simulink model "elevator"  (R2020a)
settings: Solver=VariableStepAuto  StartTime=0.0  StopTime=inf  RelTol=1e-3
PreLoadFcn:
  | slplc.api.loadDataTypes;
undefined symbols (not defined in the file): BOOL, DINT, INT, slplc
libraries: simulink x1
(part 38 of 38)

== matlab function elevator/PLCControllerSuite/__Logic/Task/Program/__Logic/XIC46/__Format ==
  data: BlockEnable input; RungIn input; RungOut input; data input
function setBlockFormat(BlockEnable, RungIn, RungOut, data)

if data~=0 && data~=1
    error('slplc:inivalidBooleanValue', 'Invalid boolean value %d', data);
end
data = logical(data);

% set parent block colors
coder.extrinsic('slplc.utils.setBlockAppearance');
persistent lastBlockEnable lastRungIn lastRungOut lastData isInit lastAnimation lastDataShow;
if isempty(lastBlockEnable)
    lastBlockEnable = true;
end
if isempty(lastRungIn)
    lastRungIn = false;
end
if isempty(lastRungOut)
    lastRungOut = false;
end
if isempty(lastData)
    lastData = data;
end
if isempty(isInit)
    isInit = true;
else
    isInit = false;
end
if isempty(lastAnimation)
    lastAnimation = false;
end
if isempty(lastDataShow)
    lastDataShow = false;
end

[animation, dataShow] = slplc.utils.setBlockAppearance('set', '%<PLCOperandTag>', {}, {}, ...
    ' = ', {'ForegroundColor'}, ...
    isInit,  ...
    BlockEnable, lastBlockEnable, ...
    RungIn,  lastRungIn, ...
    RungOut, lastRungOut, ...
    data, lastData, ...
    lastAnimation, lastDataShow);

lastBlockEnable = BlockEnable;
lastRungIn      = RungIn;
lastRungOut     = RungOut;
lastData        = data;
lastAnimation   = animation;
lastDataShow    = dataShow;
end

== matlab function elevator/PLCControllerSuite/__Logic/Task/Program/__Logic/Junction1/__Format ==
  data: BlockEnable input; RungOut input
function setBlockFormat(BlockEnable, RungOut)
% set parent block colors
coder.extrinsic('slplc.utils.setBlockAppearance');
persistent lastBlockEnable isInit lastRungOut lastAnimation lastRungOutShow;
if isempty(lastBlockEnable)
    lastBlockEnable = true;
end

if isempty(isInit)
    isInit = true;
else
    isInit = false;
end

if isempty(lastRungOut)
    lastRungOut = RungOut;
end

if isempty(lastAnimation)
    lastAnimation = false;
end

if isempty(lastRungOutShow)
    lastRungOutShow = false;
end

[animation, dataShow] = slplc.utils.setBlockAppearance('set', '', {'black', 'black'}, {}, ...
    '', {'ForegroundColor', 'BackgroundColor'}, ...
    isInit,  ...
    BlockEnable, lastBlockEnable, ...
    RungOut,   lastRungOut, ...
    RungOut,   lastRungOut, ...
    [],    [], ...
    lastAnimation, lastRungOutShow);

lastBlockEnable     = BlockEnable;
lastRungOut         = RungOut;
lastAnimation       = animation;
lastRungOutShow     = dataShow;
end

== matlab function elevator/PLCControllerSuite/__Logic/Task/Program/__Logic/XIC47/__Format ==
  data: BlockEnable input; RungIn input; RungOut input; data input
function setBlockFormat(BlockEnable, RungIn, RungOut, data)

if data~=0 && data~=1
    error('slplc:inivalidBooleanValue', 'Invalid boolean value %d', data);
end
data = logical(data);

% set parent block colors
coder.extrinsic('slplc.utils.setBlockAppearance');
persistent lastBlockEnable lastRungIn lastRungOut lastData isInit lastAnimation lastDataShow;
if isempty(lastBlockEnable)
    lastBlockEnable = true;
end
if isempty(lastRungIn)
    lastRungIn = false;
end
if isempty(lastRungOut)
    lastRungOut = false;
end
if isempty(lastData)
    lastData = data;
end
if isempty(isInit)
    isInit = true;
else
    isInit = false;
end
if isempty(lastAnimation)
    lastAnimation = false;
end
if isempty(lastDataShow)
    lastDataShow = false;
end

[animation, dataShow] = slplc.utils.setBlockAppearance('set', '%<PLCOperandTag>', {}, {}, ...
    ' = ', {'ForegroundColor'}, ...
    isInit,  ...
    BlockEnable, lastBlockEnable, ...
    RungIn,  lastRungIn, ...
    RungOut, lastRungOut, ...
    data, lastData, ...
    lastAnimation, lastDataShow);

lastBlockEnable = BlockEnable;
lastRungIn      = RungIn;
lastRungOut     = RungOut;
lastData        = data;
lastAnimation   = animation;
lastDataShow    = dataShow;
end

== matlab function elevator/PLCControllerSuite/__Logic/Task/Program/__Logic/XIC48/__Format ==
  data: BlockEnable input; RungIn input; RungOut input; data input
function setBlockFormat(BlockEnable, RungIn, RungOut, data)

if data~=0 && data~=1
    error('slplc:inivalidBooleanValue', 'Invalid boolean value %d', data);
end
data = logical(data);

% set parent block colors
coder.extrinsic('slplc.utils.setBlockAppearance');
persistent lastBlockEnable lastRungIn lastRungOut lastData isInit lastAnimation lastDataShow;
if isempty(lastBlockEnable)
    lastBlockEnable = true;
end
if isempty(lastRungIn)
    lastRungIn = false;
end
if isempty(lastRungOut)
    lastRungOut = false;
end
if isempty(lastData)
    lastData = data;
end
if isempty(isInit)
    isInit = true;
else
    isInit = false;
end
if isempty(lastAnimation)
    lastAnimation = false;
end
if isempty(lastDataShow)
    lastDataShow = false;
end

[animation, dataShow] = slplc.utils.setBlockAppearance('set', '%<PLCOperandTag>', {}, {}, ...
    ' = ', {'ForegroundColor'}, ...
    isInit,  ...
    BlockEnable, lastBlockEnable, ...
    RungIn,  lastRungIn, ...
    RungOut, lastRungOut, ...
    data, lastData, ...
    lastAnimation, lastDataShow);

lastBlockEnable = BlockEnable;
lastRungIn      = RungIn;
lastRungOut     = RungOut;
lastData        = data;
lastAnimation   = animation;
lastDataShow    = dataShow;
end

== matlab function elevator/PLCControllerSuite/__Logic/Task/Program/__Logic/XIC49/__Format ==
  data: BlockEnable input; RungIn input; RungOut input; data input
function setBlockFormat(BlockEnable, RungIn, RungOut, data)

if data~=0 && data~=1
    error('slplc:inivalidBooleanValue', 'Invalid boolean value %d', data);
end
data = logical(data);

% set parent block colors
coder.extrinsic('slplc.utils.setBlockAppearance');
persistent lastBlockEnable lastRungIn lastRungOut lastData isInit lastAnimation lastDataShow;
if isempty(lastBlockEnable)
    lastBlockEnable = true;
end
if isempty(lastRungIn)
    lastRungIn = false;
end
if isempty(lastRungOut)
    lastRungOut = false;
end
if isempty(lastData)
    lastData = data;
end
if isempty(isInit)
    isInit = true;
else
    isInit = false;
end
if isempty(lastAnimation)
    lastAnimation = false;
end
if isempty(lastDataShow)
    lastDataShow = false;
end

[animation, dataShow] = slplc.utils.setBlockAppearance('set', '%<PLCOperandTag>', {}, {}, ...
    ' = ', {'ForegroundColor'}, ...
    isInit,  ...
    BlockEnable, lastBlockEnable, ...
    RungIn,  lastRungIn, ...
    RungOut, lastRungOut, ...
    data, lastData, ...
    lastAnimation, lastDataShow);

lastBlockEnable = BlockEnable;
lastRungIn      = RungIn;
lastRungOut     = RungOut;
lastData        = data;
lastAnimation   = animation;
lastDataShow    = dataShow;
end

== matlab function elevator/PLCControllerSuite/__Logic/Task/Program/__Logic/XIC50/__Format ==
  data: BlockEnable input; RungIn input; RungOut input; data input
function setBlockFormat(BlockEnable, RungIn, RungOut, data)

if data~=0 && data~=1
    error('slplc:inivalidBooleanValue', 'Invalid boolean value %d', data);
end
data = logical(data);

% set parent block colors
coder.extrinsic('slplc.utils.setBlockAppearance');
persistent lastBlockEnable lastRungIn lastRungOut lastData isInit lastAnimation lastDataShow;
if isempty(lastBlockEnable)
    lastBlockEnable = true;
end
if isempty(lastRungIn)
    lastRungIn = false;
end
if isempty(lastRungOut)
    lastRungOut = false;
end
if isempty(lastData)
    lastData = data;
end
if isempty(isInit)
    isInit = true;
else
    isInit = false;
end
if isempty(lastAnimation)
    lastAnimation = false;
end
if isempty(lastDataShow)
    lastDataShow = false;
end

[animation, dataShow] = slplc.utils.setBlockAppearance('set', '%<PLCOperandTag>', {}, {}, ...
    ' = ', {'ForegroundColor'}, ...
    isInit,  ...
    BlockEnable, lastBlockEnable, ...
    RungIn,  lastRungIn, ...
    RungOut, lastRungOut, ...
    data, lastData, ...
    lastAnimation, lastDataShow);

lastBlockEnable = BlockEnable;
lastRungIn      = RungIn;
lastRungOut     = RungOut;
lastData        = data;
lastAnimation   = animation;
lastDataShow    = dataShow;
end

== matlab function elevator/PLCControllerSuite/__Logic/Task/Program/__Logic/XIC51/__Format ==
  data: BlockEnable input; RungIn input; RungOut input; data input
function setBlockFormat(BlockEnable, RungIn, RungOut, data)

if data~=0 && data~=1
    error('slplc:inivalidBooleanValue', 'Invalid boolean value %d', data);
end
data = logical(data);

% set parent block colors
coder.extrinsic('slplc.utils.setBlockAppearance');
persistent lastBlockEnable lastRungIn lastRungOut lastData isInit lastAnimation lastDataShow;
if isempty(lastBlockEnable)
    lastBlockEnable = true;
end
if isempty(lastRungIn)
    lastRungIn = false;
end
if isempty(lastRungOut)
    lastRungOut = false;
end
if isempty(lastData)
    lastData = data;
end
if isempty(isInit)
    isInit = true;
else
    isInit = false;
end
if isempty(lastAnimation)
    lastAnimation = false;
end
if isempty(lastDataShow)
    lastDataShow = false;
end

[animation, dataShow] = slplc.utils.setBlockAppearance('set', '%<PLCOperandTag>', {}, {}, ...
    ' = ', {'ForegroundColor'}, ...
    isInit,  ...
    BlockEnable, lastBlockEnable, ...
    RungIn,  lastRungIn, ...
    RungOut, lastRungOut, ...
    data, lastData, ...
    lastAnimation, lastDataShow);

lastBlockEnable = BlockEnable;
lastRungIn      = RungIn;
lastRungOut     = RungOut;
lastData        = data;
lastAnimation   = animation;
lastDataShow    = dataShow;
end

== matlab function elevator/PLCControllerSuite/__Logic/Task/Program/__Logic/XIC52/__Format ==
  data: BlockEnable input; RungIn input; RungOut input; data input
function setBlockFormat(BlockEnable, RungIn, RungOut, data)

if data~=0 && data~=1
    error('slplc:inivalidBooleanValue', 'Invalid boolean value %d', data);
end
data = logical(data);

% set parent block colors
coder.extrinsic('slplc.utils.setBlockAppearance');
persistent lastBlockEnable lastRungIn lastRungOut lastData isInit lastAnimation lastDataShow;
if isempty(lastBlockEnable)
    lastBlockEnable = true;
end
if isempty(lastRungIn)
    lastRungIn = false;
end
if isempty(lastRungOut)
    lastRungOut = false;
end
if isempty(lastData)
    lastData = data;
end
if isempty(isInit)
    isInit = true;
else
    isInit = false;
end
if isempty(lastAnimation)
    lastAnimation = false;
end
if isempty(lastDataShow)
    lastDataShow = false;
end

[animation, dataShow] = slplc.utils.setBlockAppearance('set', '%<PLCOperandTag>', {}, {}, ...
    ' = ', {'ForegroundColor'}, ...
    isInit,  ...
    BlockEnable, lastBlockEnable, ...
    RungIn,  lastRungIn, ...
    RungOut, lastRungOut, ...
    data, lastData, ...
    lastAnimation, lastDataShow);

lastBlockEnable = BlockEnable;
lastRungIn      = RungIn;
lastRungOut     = RungOut;
lastData        = data;
lastAnimation   = animation;
lastDataShow    = dataShow;
end

== matlab function elevator/PLCControllerSuite/__Logic/Task/Program/__Logic/XIC53/__Format ==
  data: BlockEnable input; RungIn input; RungOut input; data input
function setBlockFormat(BlockEnable, RungIn, RungOut, data)

if data~=0 && data~=1
    error('slplc:inivalidBooleanValue', 'Invalid boolean value %d', data);
end
data = logical(data);

% set parent block colors
coder.extrinsic('slplc.utils.setBlockAppearance');
persistent lastBlockEnable lastRungIn lastRungOut lastData isInit lastAnimation lastDataShow;
if isempty(lastBlockEnable)
    lastBlockEnable = true;
end
if isempty(lastRungIn)
    lastRungIn = false;
end
if isempty(lastRungOut)
    lastRungOut = false;
end
if isempty(lastData)
    lastData = data;
end
if isempty(isInit)
    isInit = true;
else
    isInit = false;
end
if isempty(lastAnimation)
    lastAnimation = false;
end
if isempty(lastDataShow)
    lastDataShow = false;
end

[animation, dataShow] = slplc.utils.setBlockAppearance('set', '%<PLCOperandTag>', {}, {}, ...
    ' = ', {'ForegroundColor'}, ...
    isInit,  ...
    BlockEnable, lastBlockEnable, ...
    RungIn,  lastRungIn, ...
    RungOut, lastRungOut, ...
    data, lastData, ...
    lastAnimation, lastDataShow);

lastBlockEnable = BlockEnable;
lastRungIn      = RungIn;
lastRungOut     = RungOut;
lastData        = data;
lastAnimation   = animation;
lastDataShow    = dataShow;
end

== matlab function elevator/PLCControllerSuite/__Logic/Task/Program/__Logic/XIC54/__Format ==
  data: BlockEnable input; RungIn input; RungOut input; data input
function setBlockFormat(BlockEnable, RungIn, RungOut, data)

if data~=0 && data~=1
    error('slplc:inivalidBooleanValue', 'Invalid boolean value %d', data);
end
data = logical(data);

% set parent block colors
coder.extrinsic('slplc.utils.setBlockAppearance');
persistent lastBlockEnable lastRungIn lastRungOut lastData isInit lastAnimation lastDataShow;
if isempty(lastBlockEnable)
    lastBlockEnable = true;
end
if isempty(lastRungIn)
    lastRungIn = false;
end
if isempty(lastRungOut)
    lastRungOut = false;
end
if isempty(lastData)
    lastData = data;
end
if isempty(isInit)
    isInit = true;
else
    isInit = false;
end
if isempty(lastAnimation)
    lastAnimation = false;
end
if isempty(lastDataShow)
    lastDataShow = false;
end

[animation, dataShow] = slplc.utils.setBlockAppearance('set', '%<PLCOperandTag>', {}, {}, ...
    ' = ', {'ForegroundColor'}, ...
    isInit,  ...
    BlockEnable, lastBlockEnable, ...
    RungIn,  lastRungIn, ...
    RungOut, lastRungOut, ...
    data, lastData, ...
    lastAnimation, lastDataShow);

lastBlockEnable = BlockEnable;
lastRungIn      = RungIn;
lastRungOut     = RungOut;
lastData        = data;
lastAnimation   = animation;
lastDataShow    = dataShow;
end

== matlab function elevator/PLCControllerSuite/__Logic/Task/Program/__Logic/XIC4/__Format ==
  data: BlockEnable input; RungIn input; RungOut input; data input
function setBlockFormat(BlockEnable, RungIn, RungOut, data)

if data~=0 && data~=1
    error('slplc:inivalidBooleanValue', 'Invalid boolean value %d', data);
end
data = logical(data);

% set parent block colors
coder.extrinsic('slplc.utils.setBlockAppearance');
persistent lastBlockEnable lastRungIn lastRungOut lastData isInit lastAnimation lastDataShow;
if isempty(lastBlockEnable)
    lastBlockEnable = true;
end
if isempty(lastRungIn)
    lastRungIn = false;
end
if isempty(lastRungOut)
    lastRungOut = false;
end
if isempty(lastData)
    lastData = data;
end
if isempty(isInit)
    isInit = true;
else
    isInit = false;
end
if isempty(lastAnimation)
    lastAnimation = false;
end
if isempty(lastDataShow)
    lastDataShow = false;
end

[animation, dataShow] = slplc.utils.setBlockAppearance('set', '%<PLCOperandTag>', {}, {}, ...
    ' = ', {'ForegroundColor'}, ...
    isInit,  ...
    BlockEnable, lastBlockEnable, ...
    RungIn,  lastRungIn, ...
    RungOut, lastRungOut, ...
    data, lastData, ...
    lastAnimation, lastDataShow);

lastBlockEnable = BlockEnable;
lastRungIn      = RungIn;
lastRungOut     = RungOut;
lastData        = data;
lastAnimation   = animation;
lastDataShow    = dataShow;
end

== matlab function elevator/PLCControllerSuite/__Logic/Task/Program/__Logic/XIC55/__Format ==
  data: BlockEnable input; RungIn input; RungOut input; data input
function setBlockFormat(BlockEnable, RungIn, RungOut, data)

if data~=0 && data~=1
    error('slplc:inivalidBooleanValue', 'Invalid boolean value %d', data);
end
data = logical(data);

% set parent block colors
coder.extrinsic('slplc.utils.setBlockAppearance');
persistent lastBlockEnable lastRungIn lastRungOut lastData isInit lastAnimation lastDataShow;
if isempty(lastBlockEnable)
    lastBlockEnable = true;
end
if isempty(lastRungIn)
    lastRungIn = false;
end
if isempty(lastRungOut)
    lastRungOut = false;
end
if isempty(lastData)
    lastData = data;
end
if isempty(isInit)
    isInit = true;
else
    isInit = false;
end
if isempty(lastAnimation)
    lastAnimation = false;
end
if isempty(lastDataShow)
    lastDataShow = false;
end

[animation, dataShow] = slplc.utils.setBlockAppearance('set', '%<PLCOperandTag>', {}, {}, ...
    ' = ', {'ForegroundColor'}, ...
    isInit,  ...
    BlockEnable, lastBlockEnable, ...
    RungIn,  lastRungIn, ...
    RungOut, lastRungOut, ...
    data, lastData, ...
    lastAnimation, lastDataShow);

lastBlockEnable = BlockEnable;
lastRungIn      = RungIn;
lastRungOut     = RungOut;
lastData        = data;
lastAnimation   = animation;
lastDataShow    = dataShow;
end

== matlab function elevator/PLCControllerSuite/__Logic/Task/Program/__Logic/XIC56/__Format ==
  data: BlockEnable input; RungIn input; RungOut input; data input
function setBlockFormat(BlockEnable, RungIn, RungOut, data)

if data~=0 && data~=1
    error('slplc:inivalidBooleanValue', 'Invalid boolean value %d', data);
end
data = logical(data);

% set parent block colors
coder.extrinsic('slplc.utils.setBlockAppearance');
persistent lastBlockEnable lastRungIn lastRungOut lastData isInit lastAnimation lastDataShow;
if isempty(lastBlockEnable)
    lastBlockEnable = true;
end
if isempty(lastRungIn)
    lastRungIn = false;
end
if isempty(lastRungOut)
    lastRungOut = false;
end
if isempty(lastData)
    lastData = data;
end
if isempty(isInit)
    isInit = true;
else
    isInit = false;
end
if isempty(lastAnimation)
    lastAnimation = false;
end
if isempty(lastDataShow)
    lastDataShow = false;
end

[animation, dataShow] = slplc.utils.setBlockAppearance('set', '%<PLCOperandTag>', {}, {}, ...
    ' = ', {'ForegroundColor'}, ...
    isInit,  ...
    BlockEnable, lastBlockEnable, ...
    RungIn,  lastRungIn, ...
    RungOut, lastRungOut, ...
    data, lastData, ...
    lastAnimation, lastDataShow);

lastBlockEnable = BlockEnable;
lastRungIn      = RungIn;
lastRungOut     = RungOut;
lastData        = data;
lastAnimation   = animation;
lastDataShow    = dataShow;
end

== matlab function elevator/PLCControllerSuite/__Logic/Task/Program/__Logic/XIO27/__Format ==
  data: BlockEnable input; RungIn input; RungOut input; data input
function setBlockFormat(BlockEnable, RungIn, RungOut, data)

if data~=0 && data~=1
    error('slplc:inivalidBooleanValue', 'Invalid boolean value %d', data);
end
data = logical(data);

% set parent block colors
coder.extrinsic('slplc.utils.setBlockAppearance');
persistent lastBlockEnable lastRungIn lastRungOut lastData isInit lastAnimation lastDataShow;
if isempty(lastBlockEnable)
    lastBlockEnable = true;
end
if isempty(lastRungIn)
    lastRungIn = false;
end
if isempty(lastRungOut)
    lastRungOut = false;
end
if isempty(lastData)
    lastData = data;
end
if isempty(isInit)
    isInit = true;
else
    isInit = false;
end
if isempty(lastAnimation)
    lastAnimation = false;
end
if isempty(lastDataShow)
    lastDataShow = false;
end

[animation, dataShow] = slplc.utils.setBlockAppearance('set', '%<PLCOperandTag>', {}, {}, ...
    ' = ', {'ForegroundColor'}, ...
    isInit,  ...
    BlockEnable, lastBlockEnable, ...
    RungIn,  lastRungIn, ...
    RungOut, lastRungOut, ...
    data, lastData, ...
    lastAnimation, lastDataShow);

lastBlockEnable = BlockEnable;
lastRungIn      = RungIn;
lastRungOut     = RungOut;
lastData        = data;
lastAnimation   = animation;
lastDataShow    = dataShow;
end

== matlab function elevator/PLCControllerSuite/__Logic/Task/Program/__Logic/OTE8/__Format ==
  data: BlockEnable input; RungIn input; RungOut input; data input
function setBlockFormat(BlockEnable, RungIn, RungOut, data)

if data~=0 && data~=1
    error('slplc:inivalidBooleanValue', 'Invalid boolean value %d', data);
end
data = logical(data);

% set parent block colors
coder.extrinsic('slplc.utils.setBlockAppearance');
persistent lastBlockEnable lastRungIn lastRungOut lastData isInit lastAnimation lastDataShow;
if isempty(lastBlockEnable)
    lastBlockEnable = true;
end
if isempty(lastRungIn)
    lastRungIn = false;
end
if isempty(lastRungOut)
    lastRungOut = false;
end
if isempty(lastData)
    lastData = data;
end
if isempty(isInit)
    isInit = true;
else
    isInit = false;
end
if isempty(lastAnimation)
    lastAnimation = false;
end
if isempty(lastDataShow)
    lastDataShow = false;
end

[animation, dataShow] = slplc.utils.setBlockAppearance('set', '%<PLCOperandTag>', {}, {}, ...
    ' = ', {'ForegroundColor'}, ...
    isInit,  ...
    BlockEnable, lastBlockEnable, ...
    RungIn,  lastRungIn, ...
    RungOut, lastRungOut, ...
    data, lastData, ...
    lastAnimation, lastDataShow);

lastBlockEnable = BlockEnable;
lastRungIn      = RungIn;
lastRungOut     = RungOut;
lastData        = data;
lastAnimation   = animation;
lastDataShow    = dataShow;
end

== matlab function elevator/PLCControllerSuite/__Logic/Task/Program/__Logic/XIC34/__Format ==
  data: BlockEnable input; RungIn input; RungOut input; data input
function setBlockFormat(BlockEnable, RungIn, RungOut, data)

if data~=0 && data~=1
    error('slplc:inivalidBooleanValue', 'Invalid boolean value %d', data);
end
data = logical(data);

% set parent block colors
coder.extrinsic('slplc.utils.setBlockAppearance');
persistent lastBlockEnable lastRungIn lastRungOut lastData isInit lastAnimation lastDataShow;
if isempty(lastBlockEnable)
    lastBlockEnable = true;
end
if isempty(lastRungIn)
    lastRungIn = false;
end
if isempty(lastRungOut)
    lastRungOut = false;
end
if isempty(lastData)
    lastData = data;
end
if isempty(isInit)
    isInit = true;
else
    isInit = false;
end
if isempty(lastAnimation)
    lastAnimation = false;
end
if isempty(lastDataShow)
    lastDataShow = false;
end

[animation, dataShow] = slplc.utils.setBlockAppearance('set', '%<PLCOperandTag>', {}, {}, ...
    ' = ', {'ForegroundColor'}, ...
    isInit,  ...
    BlockEnable, lastBlockEnable, ...
    RungIn,  lastRungIn, ...
    RungOut, lastRungOut, ...
    data, lastData, ...
    lastAnimation, lastDataShow);

lastBlockEnable = BlockEnable;
lastRungIn      = RungIn;
lastRungOut     = RungOut;
lastData        = data;
lastAnimation   = animation;
lastDataShow    = dataShow;
end

== matlab function elevator/PLCControllerSuite/__Logic/Task/Program/__Logic/Variable Write1/__Format ==
  data: data input
function setBlockFormat(data)
% set parent block colors
coder.extrinsic('slplc.utils.setBlockAppearance');
persistent isInit lastData  lastAnimation lastDataShow;

if isempty(isInit)
    isInit = true;
else
    isInit = false;
end

if isempty(lastData)
    lastData = data;
end

if isempty(lastAnimation)
    lastAnimation = false;
end

if isempty(lastDataShow)
    lastDataShow = false;
end

[animation, dataShow] = slplc.utils.setBlockAppearance('set', '', {}, {}, ...
    '%<PLCOperandTag> = ', {}, ...
    isInit,  ...
    true,  true, ...
    false, false, ...
    false, false, ...
    data,  lastData, ...
    lastAnimation, lastDataShow);

lastData        = data;
lastAnimation   = animation;
lastDataShow    = dataShow;
end

== matlab function elevator/PLCControllerSuite/__Logic/Task/Program/__Logic/Variable Write2/__Format ==
  data: data input
function setBlockFormat(data)
% set parent block colors
coder.extrinsic('slplc.utils.setBlockAppearance');
persistent isInit lastData  lastAnimation lastDataShow;

if isempty(isInit)
    isInit = true;
else
    isInit = false;
end

if isempty(lastData)
    lastData = data;
end

if isempty(lastAnimation)
    lastAnimation = false;
end

if isempty(lastDataShow)
    lastDataShow = false;
end

[animation, dataShow] = slplc.utils.setBlockAppearance('set', '', {}, {}, ...
    '%<PLCOperandTag> = ', {}, ...
    isInit,  ...
    true,  true, ...
    false, false, ...
    false, false, ...
    data,  lastData, ...
    lastAnimation, lastDataShow);

lastData        = data;
lastAnimation   = animation;
lastDataShow    = dataShow;
end

== matlab function elevator/PLCControllerSuite/__Logic/Task/Program/__Logic/Variable Write3/__Format ==
  data: data input
function setBlockFormat(data)
% set parent block colors
coder.extrinsic('slplc.utils.setBlockAppearance');
persistent isInit lastData  lastAnimation lastDataShow;

if isempty(isInit)
    isInit = true;
else
    isInit = false;
end

if isempty(lastData)
    lastData = data;
end

if isempty(lastAnimation)
    lastAnimation = false;
end

if isempty(lastDataShow)
    lastDataShow = false;
end

[animation, dataShow] = slplc.utils.setBlockAppearance('set', '', {}, {}, ...
    '%<PLCOperandTag> = ', {}, ...
    isInit,  ...
    true,  true, ...
    false, false, ...
    false, false, ...
    data,  lastData, ...
    lastAnimation, lastDataShow);

lastData        = data;
lastAnimation   = animation;
lastDataShow    = dataShow;
end

== matlab function elevator/PLCControllerSuite/__Logic/Task/Program/__Logic/XIC41/__Format ==
  data: BlockEnable input; RungIn input; RungOut input; data input
function setBlockFormat(BlockEnable, RungIn, RungOut, data)

if data~=0 && data~=1
    error('slplc:inivalidBooleanValue', 'Invalid boolean value %d', data);
end
data = logical(data);

% set parent block colors
coder.extrinsic('slplc.utils.setBlockAppearance');
persistent lastBlockEnable lastRungIn lastRungOut lastData isInit lastAnimation lastDataShow;
if isempty(lastBlockEnable)
    lastBlockEnable = true;
end
if isempty(lastRungIn)
    lastRungIn = false;
end
if isempty(lastRungOut)
    lastRungOut = false;
end
if isempty(lastData)
    lastData = data;
end
if isempty(isInit)
    isInit = true;
else
    isInit = false;
end
if isempty(lastAnimation)
    lastAnimation = false;
end
if isempty(lastDataShow)
    lastDataShow = false;
end

[animation, dataShow] = slplc.utils.setBlockAppearance('set', '%<PLCOperandTag>', {}, {}, ...
    ' = ', {'ForegroundColor'}, ...
    isInit,  ...
    BlockEnable, lastBlockEnable, ...
    RungIn,  lastRungIn, ...
    RungOut, lastRungOut, ...
    data, lastData, ...
    lastAnimation, lastDataShow);

lastBlockEnable = BlockEnable;
lastRungIn      = RungIn;
lastRungOut     = RungOut;
lastData        = data;
lastAnimation   = animation;
lastDataShow    = dataShow;
end

== matlab function elevator/PLCControllerSuite/__Logic/Task/Program/__Logic/TON/Instruction_Enable/__Logic ==
  data: EN output; TT output; RungIn input; PRE input; EN input; DN input; DN output; ACC output; ACC input; currentTime input; lastTime input
function [EN, TT, DN, ACC]  = TON(RungIn, PRE, EN, DN, ACC, currentTime, lastTime)
% TON algorithm

if RungIn
    % Rung-condition-in is True
    if PRE < 0 || ACC < 0
        error('slplc:TONError', '.PRE or .ACC cannot be negtive values');
    end
    TT = true;
    if ~DN
        if EN
            deltaT = currentTime - lastTime;
            ACC = ACC + cast(deltaT, class(ACC));
            if ACC == intmax(class(ACC)) || ACC >= PRE
                TT = false;
                DN = true;
            end
        end
    else
        TT = false;
    end
    EN = true;
    % True end
else
    % Rung-condition-in is False
    EN    = false;
    TT    = false;
    DN    = false;
    ACC   = cast(0, class(ACC));
    % False end
end

end

== matlab function elevator/PLCControllerSuite/__Logic/Task/Program/__Logic/OTE1/__Format ==
  data: BlockEnable input; RungIn input; RungOut input; data input
function setBlockFormat(BlockEnable, RungIn, RungOut, data)

if data~=0 && data~=1
    error('slplc:inivalidBooleanValue', 'Invalid boolean value %d', data);
end
data = logical(data);

% set parent block colors
coder.extrinsic('slplc.utils.setBlockAppearance');
persistent lastBlockEnable lastRungIn lastRungOut lastData isInit lastAnimation lastDataShow;
if isempty(lastBlockEnable)
    lastBlockEnable = true;
end
if isempty(lastRungIn)
    lastRungIn = false;
end
if isempty(lastRungOut)
    lastRungOut = false;
end
if isempty(lastData)
    lastData = data;
end
if isempty(isInit)
    isInit = true;
else
    isInit = false;
end
if isempty(lastAnimation)
    lastAnimation = false;
end
if isempty(lastDataShow)
    lastDataShow = false;
end

[animation, dataShow] = slplc.utils.setBlockAppearance('set', '%<PLCOperandTag>', {}, {}, ...
    ' = ', {'ForegroundColor'}, ...
    isInit,  ...
    BlockEnable, lastBlockEnable, ...
    RungIn,  lastRungIn, ...
    RungOut, lastRungOut, ...
    data, lastData, ...
    lastAnimation, lastDataShow);

lastBlockEnable = BlockEnable;
lastRungIn      = RungIn;
lastRungOut     = RungOut;
lastData        = data;
lastAnimation   = animation;
lastDataShow    = dataShow;
end

== matlab function elevator/PLCControllerSuite/__Logic/Task/Program/__Logic/TON/__Format ==
  data: BlockEnable input; RungIn input; RungOut input; data input
function setBlockFormat(BlockEnable, RungIn, RungOut, data)
% set parent block colors
coder.extrinsic('slplc.utils.setBlockAppearance');
persistent lastBlockEnable lastRungIn lastRungOut lastData isInit lastAnimation lastDataShow;
if isempty(lastBlockEnable)
    lastBlockEnable = true;
end
if isempty(lastRungIn)
    lastRungIn = false;
end
if isempty(lastRungOut)
    lastRungOut = false;
end
if isempty(lastData)
    lastData = data;
end
if isempty(isInit)
    isInit = true;
else
    isInit = false;
end
if isempty(lastAnimation)
    lastAnimation = false;
end
if isempty(lastDataShow)
    lastDataShow = false;
end

[animation, dataShow] = slplc.utils.setBlockAppearance('set', '%<PLCBlockType>: %<PLCOperandTag>', {}, {}, ...
    ' = ', {'ForegroundColor'}, ...
    isInit,  ...
    BlockEnable, lastBlockEnable, ...
    RungIn,  lastRungIn, ...
    RungOut, lastRungOut, ...
    data, lastData, ...
    lastAnimation, lastDataShow);

lastBlockEnable = BlockEnable;
lastRungIn      = RungIn;
lastRungOut     = RungOut;
lastData        = data;
lastAnimation   = animation;
lastDataShow    = dataShow;
end

== matlab function elevator/PLCControllerSuite/__Logic/Task/Program/__Logic/OTE11/__Format ==
  data: BlockEnable input; RungIn input; RungOut input; data input
function setBlockFormat(BlockEnable, RungIn, RungOut, data)

if data~=0 && data~=1
    error('slplc:inivalidBooleanValue', 'Invalid boolean value %d', data);
end
data = logical(data);

% set parent block colors
coder.extrinsic('slplc.utils.setBlockAppearance');
persistent lastBlockEnable lastRungIn lastRungOut lastData isInit lastAnimation lastDataShow;
if isempty(lastBlockEnable)
    lastBlockEnable = true;
end
if isempty(lastRungIn)
    lastRungIn = false;
end
if isempty(lastRungOut)
    lastRungOut = false;
end
if isempty(lastData)
    lastData = data;
end
if isempty(isInit)
    isInit = true;
else
    isInit = false;
end
if isempty(lastAnimation)
    lastAnimation = false;
end
if isempty(lastDataShow)
    lastDataShow = false;
end

[animation, dataShow] = slplc.utils.setBlockAppearance('set', '%<PLCOperandTag>', {}, {}, ...
    ' = ', {'ForegroundColor'}, ...
    isInit,  ...
    BlockEnable, lastBlockEnable, ...
    RungIn,  lastRungIn, ...
    RungOut, lastRungOut, ...
    data, lastData, ...
    lastAnimation, lastDataShow);

lastBlockEnable = BlockEnable;
lastRungIn      = RungIn;
lastRungOut     = RungOut;
lastData        = data;
lastAnimation   = animation;
lastDataShow    = dataShow;
end

== matlab function elevator/PLCControllerSuite/__Logic/Task/Program/__Logic/XIC38/__Format ==
  data: BlockEnable input; RungIn input; RungOut input; data input
function setBlockFormat(BlockEnable, RungIn, RungOut, data)

if data~=0 && data~=1
    error('slplc:inivalidBooleanValue', 'Invalid boolean value %d', data);
end
data = logical(data);

% set parent block colors
coder.extrinsic('slplc.utils.setBlockAppearance');
persistent lastBlockEnable lastRungIn lastRungOut lastData isInit lastAnimation lastDataShow;
if isempty(lastBlockEnable)
    lastBlockEnable = true;
end
if isempty(lastRungIn)
    lastRungIn = false;
end
if isempty(lastRungOut)
    lastRungOut = false;
end
if isempty(lastData)
    lastData = data;
end
if isempty(isInit)
    isInit = true;
else
    isInit = false;
end
if isempty(lastAnimation)
    lastAnimation = false;
end
if isempty(lastDataShow)
    lastDataShow = false;
end

[animation, dataShow] = slplc.utils.setBlockAppearance('set', '%<PLCOperandTag>', {}, {}, ...
    ' = ', {'ForegroundColor'}, ...
    isInit,  ...
    BlockEnable, lastBlockEnable, ...
    RungIn,  lastRungIn, ...
    RungOut, lastRungOut, ...
    data, lastData, ...
    lastAnimation, lastDataShow);

lastBlockEnable = BlockEnable;
lastRungIn      = RungIn;
lastRungOut     = RungOut;
lastData        = data;
lastAnimation   = animation;
lastDataShow    = dataShow;
end

== matlab function elevator/PLCControllerSuite/__Logic/Task/Program/__Logic/XIC39/__Format ==
  data: BlockEnable input; RungIn input; RungOut input; data input
function setBlockFormat(BlockEnable, RungIn, RungOut, data)

if data~=0 && data~=1
    error('slplc:inivalidBooleanValue', 'Invalid boolean value %d', data);
end
data = logical(data);

% set parent block colors
coder.extrinsic('slplc.utils.setBlockAppearance');
persistent lastBlockEnable lastRungIn lastRungOut lastData isInit lastAnimation lastDataShow;
if isempty(lastBlockEnable)
    lastBlockEnable = true;
end
if isempty(lastRungIn)
    lastRungIn = false;
end
if isempty(lastRungOut)
    lastRungOut = false;
end
if isempty(lastData)
    lastData = data;
end
if isempty(isInit)
    isInit = true;
else
    isInit = false;
end
if isempty(lastAnimation)
    lastAnimation = false;
end
if isempty(lastDataShow)
    lastDataShow = false;
end

[animation, dataShow] = slplc.utils.setBlockAppearance('set', '%<PLCOperandTag>', {}, {}, ...
    ' = ', {'ForegroundColor'}, ...
    isInit,  ...
    BlockEnable, lastBlockEnable, ...
    RungIn,  lastRungIn, ...
    RungOut, lastRungOut, ...
    data, lastData, ...
    lastAnimation, lastDataShow);

lastBlockEnable = BlockEnable;
lastRungIn      = RungIn;
lastRungOut     = RungOut;
lastData        = data;
lastAnimation   = animation;
lastDataShow    = dataShow;
end
